simulink model "Candidacy_Exam_RR"  (R2023a)
settings: Solver=VariableStepAuto  StartTime=0  StopTime=1000  FixedStep=0.01  RelTol=1e-3
model workspace (MAT data in the model file):
  finalint = 0
  firstWarning = 1
  originalScenarioChecksum = '114339432DE22364D47BB28FC96DC10C'
undefined symbols (not defined in the file): Acceleration, ActorID, AngularVelocity, curvature, DefaultGear, Defined, DEND_B, DEND_S, DEND_T, direction, DiscIntNeverNeededParam, driving, Ego, EgoRefPose, gradbp, L, Lane, LF, LR, m, matlabshared, MAX_BRAKE, MAX_STEER, MAX_TORQUE, maxNumActors, MCAR, MIN_BRAKE, MIN_STEER, MIN_TORQUE, n, NUMD_B, NUMD_S, NUMD_T, Pitch, Pose, Position, psi_o, R, Roll, RRdamp, SceneInfo, session, sigbuilder_block, STEER_RATIO, stopSign_ID, Tdead, thetaRefs, TL_ID, TrackWidth, Ts, ts, User, Vdead, Velocity, WB, X_o, xRef2s, Y_o, Yaw, yRef2s
libraries: drivingscenarioandsensors x13, roadrunnerscenario x11, simulink x8, simulink_extras x5, drivingvehiclecontroller x2, trackingutilitieslib x2, robotalgslib x1, mpcadaslib x1, slpidlib x1, drivinglib x1, autolibshared x1, vehdynlibviscommon x1
(part 5 of 5)

== stateflow chart Candidacy_Exam_RR/Behavioural Planner/Chart ==
  settings: updateMethod=DISCRETE  sampleTime=Ts
  state Stationary
    en,du:
    VelCmd = 0;
    CurrentVelCmd = VelCmd;
    Navi = 0;
    Trans = 0;
    StopSim = 0;
    Tgap = 1;
    HoldBrake = 1;
    Braking = 0;
  state Navigation
    state RailCrossing [commented out]
      state Stop [commented out]
        en:
        VelCmd = 0;
        Braking = 1;
        CurrentVelCmd = VelCmd;
      state Approaching [commented out]
        en:
        Braking = 1;
        Tgap = 0;
        Trans = 0;
      state Transition [commented out]
        en:
        Tgap = 1;
        Trans = 1;
        Braking = 0;
        VelCmd = SceneSpeed;
        CurrentVelCmd = VelCmd;
      state ExitScene [commented out]
        en:
        ExitFlag = 1;
      (default) -> Navigation.RailCrossing.Approaching [commented out]
      Navigation.RailCrossing.Approaching -> Navigation.RailCrossing.Stop [commented out] : [D2S <= 6 && (RRCross == 1 || ObjectDist <= TransDist)]
      Navigation.RailCrossing.Transition -> Navigation.RailCrossing.Approaching [commented out] : [ObjectDist <= TransDist]
      Navigation.RailCrossing.Approaching -> Navigation.RailCrossing.Transition [commented out] : [RRCross == 0 && ObjectDist > TransDist && D2S <= 6]
      Navigation.RailCrossing.Stop -> Navigation.RailCrossing.Transition [commented out] : [RRCross == 0 && ObjectDist > TransDist]
      Navigation.RailCrossing.Approaching -> Navigation.RailCrossing.ExitScene [commented out] : [SceneID ~= 10]
      Navigation.RailCrossing.Transition -> Navigation.RailCrossing.ExitScene [commented out] : [SceneID == 0]
    state RoundAbout
      state Approaching
        en:
        Braking = 1;
        Trans = 0;
        Tgap = 0;
      state Stop
        en:
        VelCmd = 0;
        Braking = 1;
        CurrentVelCmd = VelCmd;
      state ExitScene
        en:
        ExitFlag = 1;
      state Transition
        en:
        Tgap = 1;
        Trans = 1;
        Braking = 0;
        VelCmd = SceneSpeed;
        CurrentVelCmd = VelCmd;
      (default) -> Navigation.RoundAbout.Approaching
      Navigation.RoundAbout.Approaching -> Navigation.RoundAbout.Stop [order 1] : [D2S <= 6]
      Navigation.RoundAbout.Stop -> Navigation.RoundAbout.Transition : [Clear2Go == 1]
      Navigation.RoundAbout.Approaching -> Navigation.RoundAbout.ExitScene [order 2] : [SceneID ~= 9]
      Navigation.RoundAbout.Transition -> Navigation.RoundAbout.ExitScene : [SceneID == 0]
    state DestCheck
      en,du:
      % dest reached?
      (default) -> (junction 47)
      (junction 47) -> (junction 48) [order 1] : [D2D < 2]
      (junction 47) -> (junction 49) [order 2] : {DestReached = 0;}
      (junction 48) -> (junction 50) : {DestReached = 1;}
      (junction 50) -> (junction 49) : {StopSim = 1;}
      (junction 49) -> (junction 51)
    state TrafficLight [commented out]
      note: Yellow light duration is 1s
      state Stop [commented out]
        en:
        Braking = 1;
        VelCmd = 0;
        CurrentVelCmd = VelCmd;
      state Approaching [commented out]
        en:
        Tgap = 0;
        Trans = 0;
        T2S = 0;
        %if TLstate(1,4) == 1
        Braking = 1;
        %else
        % ACC = 0;
        %end
      state DecisionOnYellow [commented out]
        en:
        T2S = D2S/EgoSpeed;
      state Transition [commented out]
        en:
        Trans = 1;
        Braking = 0;
        Tgap = 1;
        VelCmd = SceneSpeed;
        CurrentVelCmd = VelCmd;
      state ExitScene [commented out]
        en:
        ExitFlag = 1;
      DecisionOnYellow -> Navigation.TrafficLight.Approaching [commented out] : [T2S > 1.2]
      (default) -> Navigation.TrafficLight.Approaching [commented out]
      Navigation.TrafficLight.Approaching -> Navigation.TrafficLight.Stop [commented out] : [D2S <= 6]
      Navigation.TrafficLight.Stop -> Navigation.TrafficLight.Transition [commented out] : [TLstate(1,4) == 3 && ObjectDist > TransDist]
      Navigation.TrafficLight.Transition -> Navigation.TrafficLight.Approaching [commented out] : [TLstate(1,4) == 1  || ObjectDist < TransDist]
      Navigation.TrafficLight.Approaching -> Navigation.TrafficLight.Transition [commented out] : [TLstate(1,4) == 3 && ObjectDist > TransDist]
      Navigation.TrafficLight.Approaching -> Navigation.TrafficLight.ExitScene [commented out] : [SceneID ~= 8]
      Navigation.TrafficLight.Transition -> DecisionOnYellow [commented out] : [TLstate(1,4) == 2]
      DecisionOnYellow -> Navigation.TrafficLight.Transition [commented out] : [T2S <= 1.2]
      Navigation.TrafficLight.Transition -> Navigation.TrafficLight.ExitScene [commented out] : [SceneID == 0]
    state Drive
      en :
      HoldBrake = 0;
      VelCmd = RoadSpeed;
      CurrentVelCmd = VelCmd;
      ExitFlag = 0;
    state Go
      en:
      VelCmd = RoadSpeed;
      CurrentVelCmd = VelCmd;
      Trans = 0;
      ExitFlag = 0;
      Braking = 0;
      HoldBrake = 1;
    state StopSign
      state StoptSign4way
        state CheckInt
          du:
          % stopped?
          % ss priority?
        state CheckSS
          % stopped?
          % ss priority?
        state Transition
          en:
          % stay here while trans?!
          % while ~crossedLimitLine of TargetLane
          Trans = 1;
          Braking = 0;
          Tgap = 1;
          VelCmd = SceneSpeed;
          CurrentVelCmd = VelCmd;
        state ExitScene
          en:
          ExitFlag = 1;
        (default) -> Navigation.StopSign.StoptSign4way.CheckSS
        Navigation.StopSign.StoptSign4way.CheckSS -> Navigation.StopSign.StoptSign4way.CheckInt : [EgoSpeed < VelStop]
        Navigation.StopSign.StoptSign4way.CheckInt -> Navigation.StopSign.StoptSign4way.Transition : [egoSSPriority == 1 && Clear2Go == 1]
        Navigation.StopSign.StoptSign4way.Transition -> Navigation.StopSign.StoptSign4way.ExitScene : [SceneID == 0 && after(2,sec)]
      state SStype
        state Approaching
          en:
          %VelCmd = ApproachingSpeed;
          Braking = 1;
          Trans = 0;
          Tgap = 0;
        state Stop
          en:
          VelCmd = 0;
          Braking = 1;
          CurrentVelCmd = VelCmd;
        Navigation.StopSign.SStype.Stop -> 410 [order 1] : [numSS == 4]
        (default) -> Navigation.StopSign.SStype.Approaching
        Navigation.StopSign.SStype.Approaching -> Navigation.StopSign.SStype.Stop : [D2S <= 15]
        Navigation.StopSign.SStype.Stop -> 414 [order 2] : [numSS == 2]
      state StopSign2way
        state CheckInt
          en:
          VelCmd = 0;
          HoldBrake = 1;
          CurrentVelCmd = VelCmd;
        state CheckSS
          % stopped?
          % ss priority?
        state Transition1
          en:
          % stay here while trans?!
          % while ~crossedLimitLine of TargetLane
          Trans = 1;
          Braking = 0;
          HoldBrake = 0;
          Tgap = 1;
          VelCmd = SceneSpeed;
          CurrentVelCmd = VelCmd;
        state ExitScene1
          en:
          ExitFlag = 1;
        (default) -> Navigation.StopSign.StopSign2way.CheckSS
        Navigation.StopSign.StopSign2way.CheckSS -> Navigation.StopSign.StopSign2way.CheckInt : [EgoSpeed < VelStop]
        Navigation.StopSign.StopSign2way.CheckInt -> Transition1 : [egoSSPriority == 1 && ToAClearance == 1]
        Transition1 -> Navigation.StopSign.StopSign2way.CheckInt [order 2] : [ToAClearance == 0]
        Transition1 -> ExitScene1 [order 1] : [SceneID == 0 && after(1,sec) && egoExit == 1]
      (default) -> SStype
      416 -> StoptSign4way
      411 -> StopSign2way
    Go -> RailCrossing [commented out] : [SceneID == 10]
    Drive -> RailCrossing [commented out] : [SceneID == 10]
    RailCrossing -> Go [commented out] : [ExitFlag == 1]
    Go -> RoundAbout [order 2] : [SceneID == 9]
    Drive -> RoundAbout [order 1] : [SceneID == 9]
    RoundAbout -> Go : [ExitFlag == 1]
    (default) -> DestCheck
    Drive -> TrafficLight [commented out] : [SceneID == 8]
    DestCheck -> Drive : [DestReached == 0]
    Go -> TrafficLight [commented out] : [SceneID == 8]
    Drive -> DestCheck [order 3] : [D2D < 2]
    TrafficLight -> Go [commented out] : [ExitFlag == 1]
    Drive -> StopSign [order 2] : [SceneID == 7]
    StopSign -> Go : [ExitFlag == 1]
    Go -> DestCheck [order 1] : [SceneID == 0]
    Go -> StopSign [order 3] : [SceneID == 7]
  (default) -> Stationary
  Stationary -> Navigation : [Navigate == 1]
  Navigation -> Stationary : [Navigate == 0 || DestReached == 1]
  data: TLstate input; numSS input; egoExit input; ToAClearance input; TransDist input; ApproachingSpeed input; EgoSpeed input; ObjectDist input; SceneSpeed input; SDist input; RRCross input; D2S input; DestReached local; Navigate input; ExitFlag local; D2D input; Clear2Go input; RoadSpeed input; CurrentVelCmd local; Navi local; VelCmd output; HoldBrake output; SceneID input; Tgap output; Trans output; StopSim output; Braking output; T2S local; VelStop input; egoSSPriority input

== matlab function Candidacy_Exam_RR/Behavioural Planner/MATLAB Function ==
  data: u input; y output
function y = fcn(u)

y = u;

== matlab function Candidacy_Exam_RR/Subsystem/Function-Call Subsystem/MATLAB Function1 ==
  data: EgoPosition input; MIOPos input; curvature input; MIOVel input; V_i input; xd output; yd output; laneL input; laneR input; V_desired input; LCinProgress output
function [xd,yd,LCinProgress] = traj(EgoPosition,MIOPos,curvature,MIOVel, V_i, laneL, laneR, V_desired)
Vx_i =0;Vx_f=0;Vy_i=0;Vy_f=0;Ax_i=0;Ax_f=0;Ay_i=0;Ay_f=0;T_i=0;T_f=0;V_f=0;A_f=0;x_set=0;y_set=0;theta4=0;

P = zeros(6,6);
% xq = zeros(1,size(RefPath,1)); yq = zeros(1,size(RefPath,2));
EgoPosition(1,2)=-EgoPosition(1,2);
x_init= EgoPosition(1,1)+2; y_init = EgoPosition(1,2)-2;
% xq = RefPath(:,1)'; 
% yq = RefPath(:,2)';
num_foc_t = 98;
V_max= V_desired; ad_n=0; vd_n=MIOVel; wd_n=vd_n*curvature;
lane_width = 3.6 * (laneL-laneR); % +1 if left of current lane and -1 if right of current lane(rahul flipped)
xd = zeros(num_foc_t+1,1); 
yd = zeros(num_foc_t+1,1);
xf =0; 
yf = 0;

    %xf = [EgoPosition(1,1)+ MIOPos(1) ]; yf = [ EgoPosition(1,2)+ MIOPos(2) + lane_width];  
    xf = [EgoPosition(1,1)+ 20 ]; yf = [EgoPosition(1,2)+ lane_width]; % 80
    V_f = V_max;
    W_f = V_f*curvature;
    A_f = 0;

    %dist2crash = sqrt((x_init-MIOPos(1))^2+(y_init-MIOPos(2))^2);
    %dist2crash = 40;
    %T_f = abs(dist2crash/(MIOVel-V_i));
    T_f = 3;
    P = [1, T_i, T_i^2, T_i^3, T_i^4, T_i^5;
         0, 1, 2*T_i, 3*T_i^2, 4*T_i^3, 5*T_i^4;
         0, 0, 2, 6*T_i, 12*T_i^2, 20*T_i^3;
         1, T_f, T_f^2, T_f^3, T_f^4, T_f^5;
         0, 1, 2*T_f, 3*T_f^2, 4*T_f^3, 5*T_f^4;
         0, 0, 2, 6*T_f, 12*T_f^2, 20*T_f^3];

%     mtang4 = (yq(1,index+2)-yq(1,index+1))/(xq(1,index+2)-xq(1,index+1));

    Vx_i = vd_n*cos(theta4); 
    Vy_i = vd_n*sin(theta4); 
    Ax_i = ad_n*cos(theta4)-vd_n*sin(theta4)*wd_n; 
    Ay_i = ad_n*sin(theta4)+vd_n*cos(theta4)*wd_n;

%     if(xq(index+2)-xq(index+1)<0)
%         theta_4 = pi + atan(mtang4);
%     else
%         theta_4 = atan(mtang4);
%     end

    theta_4 =0;
    Vx_f = V_f*cos(theta_4); % curvature angle
    Vy_f = V_f*sin(theta_4);
    Ax_f = A_f*cos(theta_4)-V_f*sin(theta_4)*W_f;
    Ay_f = A_f*sin(theta_4)+V_f*cos(theta_4)*W_f;

    g1 = [x_init; Vx_i; Ax_i; xf; Vx_f; Ax_f];
    g2 = [y_init; Vy_i; Ay_i; yf; Vy_f; Ay_f];

    a_coeff = P\g1;
    b_coeff = P\g2;
    
    td = T_i;
    scatter(x_init,y_init,'go')
    hold on; 
    scatter(xf,yf,'ro')
    hold on;
    
    for f = 1:(num_foc_t+1)
        xd(f,1) = [1,td,td^2,td^3,td^4,td^5]*a_coeff 
        yd(f,1) = [1,td,td^2,td^3,td^4,td^5]*b_coeff
        td = td + (T_f - T_i)/num_foc_t;
        scatter(xd(f,1),yd(f,1),'y.');
    end

LCinProgress = 1;

% hold on;
end

== matlab function Candidacy_Exam_RR/Behavioural Planner/StopSignPriority ==
  settings: updateMethod=DISCRETE
  data: ToAClearance output; SDist input; D2S input; ObjTracks input; egoSSPriority output; SceneTracks input; egoPose input; egoSpeed input; numSS output; VelStop input; WB input; d output; flag input; flag output; midpoint input; midpoint output; egoExit output; egoEnter input; egoEnter output
function [ToAClearance, egoSSPriority, numSS, d, flag, midpoint, egoExit, egoEnter]  = StopSignPriority(SDist, D2S, ObjTracks, SceneTracks, egoPose, egoSpeed, VelStop, WB, flag, midpoint, egoEnter)
% calculate covariance matrix outside, input to this block is modified with final, unique detections

egoPose(2) = -egoPose(2);
egoPose(3) = -egoPose(3);
persistent SSPriority C1x C2y C3x C4y
% find stop signs + one of 2way or 4way or T-junction

% find number of signs (until we reach 0 valued columns)
numSS = 0;
for j = 1:length(SceneTracks(1,:))
    if any(SceneTracks(:,j))
        numSS = numSS + 1;
    end
end

% find number of cars
numCars = 0;
for j = 1:length(ObjTracks(1,:))
    if any(ObjTracks(:,j))
        numCars = numCars + 1;
    end
end


egoSSPriority = 1;
ToAClearance = 1;
% tempPriority = zeros(numCars+1,1);
d = zeros(10, 5); % distance, velocity, time, location (wrt ego), exit (leaving ints)
Objang = zeros(10, 1);
% priorityTable = zeros(numCars+1, 5);
egoExitang = egoPose(3) - atan2d(midpoint(2)-egoPose(2),midpoint(1)-egoPose(1)); % 0 deg = straight , + = right
egoExitdist = sqrt((midpoint(2)-egoPose(2))^2+(midpoint(1)-egoPose(1))^2);

if abs(egoExitang) >= 135 && egoExitdist >= 1 && egoEnter == 1
    d(1,5) = 1; % left the ints
    egoEnter = 0;
    flag = 0;
elseif abs(egoExitang) >= 135 && egoExitdist <= 10
    d(1,5) = 1;
end
egoExit = d(1,5);


if D2S <= SDist || egoEnter == 1

    % [~, index] = min(abs(SceneTracks(1,:)'));
    if numSS > 0

        Vmd = [-egoSpeed*sind(egoPose(3)), egoSpeed*cosd(egoPose(3))];
        rot = [cosd(egoPose(3)) -sind(egoPose(3)); sind(egoPose(3)) cosd(egoPose(3))];

        % intersection region
        if flag == 0
            C1x = min(SceneTracks(1, 1:numSS)) - (WB + 3);
            C2y = min(SceneTracks(3, 1:numSS)) - (WB + 3);
            C3x = max(SceneTracks(1, 1:numSS)) + (WB + 3);
            C4y = max(SceneTracks(3, 1:numSS)) + (WB + 3);
            C1 = rot*[C1x; C2y] + egoPose(1:2)';
            C2 = rot*[C3x; C4y] + egoPose(1:2)';
            midpoint = (C1+C2)./2;
            % midpoint = [2*egoPose(1)-C4y-C2y; 2*egoPose(2)+C1x+C3x]./2;
        %   scatter(-SceneTracks(3,:)+egoPose(1),SceneTracks(1,:)+egoPose(2),'blue','filled')   
            scatter(midpoint(1), midpoint(2), 'blue', 'filled')
            rectangle('Position',[egoPose(1)-C4y egoPose(2)+C1x abs(C4y-C2y) abs(C3x-C1x)])
            flag = C1x;
        end

       
        midpoint_ego = rot'*(midpoint - egoPose(1:2)');
        % loop through num of cars (j)
    
        d(1,1) = sqrt((midpoint(1) - egoPose(1))^2 + (midpoint(2) - egoPose(2))^2);
        d(1,2) = egoSpeed;
        d(1,3) = d(1,1)/d(1,2);     %add ego TOA
        d(1,4) = 4; % 4 is the location of the ego vehicle itself
        
        if d(1,1) <= 3
            ToAThreshold = 1;
        else
            ToAThreshold = 3;
        end

        if d(1,1) <= flag
            egoEnter = 1;
        end

    
        % loop through signs (vectorized)
        % if smallest dist 
        % d(:,3) -> TOA = v/dist
    
        if numCars > 0
            for k = 1:numCars
                d(k+1,1) = sqrt((midpoint_ego(2)-ObjTracks(3,k))^2+(midpoint_ego(1)-ObjTracks(1,k))^2); %sqrt((midpoint(1) - (-ObjTracks(3,k)+egoPose(1)))^2 + (midpoint(2) - (ObjTracks(1,k)+egoPose(2)))^2); 
                d(k+1,2) = sqrt((Vmd(1) - ObjTracks(2,k))^2 + (Vmd(2) - ObjTracks(4,k))^2);
                d(k+1,3) = d(k+1,1)/d(k+1,2); % TOA of other cars
                Objang(k) = atan2d(ObjTracks(1,k), -ObjTracks(3,k));
                                
                % Identify cars location (direction) wrt ego
                if Objang(k) <= 60
                    d(k+1,4) = 1; % 1 = E, 2 = N, 3 = W
                elseif Objang(k) > 60  && Objang(k) < 120
                    d(k+1,4) = 2; % 1 = E, 2 = N, 3 = W
                elseif Objang(k) >= 120
                    d(k+1,4) = 3; % 1 = E, 2 = N, 3 = W
                end

                % Identifying leaving cars
                
                ActorHeading = atan2d(ObjTracks(2,k) - Vmd(1), -ObjTracks(4,k) - Vmd(2));
                actorExitang = ActorHeading - atan2d(midpoint_ego(1)-ObjTracks(1,k),midpoint_ego(2)+ObjTracks(3,k)); % 0 deg = straight , + = right
                %actorExitdist = sqrt((midpoint_ego(2)-ObjTracks(3,k))^2+(midpoint_ego(1)-ObjTracks(1,k))^2);
                

                if abs(actorExitang) >= 135 && d(k+1,1) >= 10 
                    d(k+1,5) = 1; % left the ints
                else
                    d(k+1,5) = 0; % did not leave
                end

    
            end
    
            if numSS == 4 
                % Assign priorities based on rank TOA #1, before vehicle stops
                % d1 = d(d(:,1)~=0,:);
                [car, SSPriority] = sort(d(d(:,1)~=0 & d(:,5)==0));
                % priorityTable(:, 1:2) = [car, priority];
        
                tempPriority = find(SSPriority == 1); % ego SS priority
                % for idx = 1:nn(vv<vv(find(nn==1)))
                % 
                % end
        
                egoSSPriority = tempPriority(1);
    
            elseif numSS == 2
                [car, SSPriority] = sort(d((d(:,4)==2 | d(:,4)==4) & d(:,5)==0));
                tempPriority = find(SSPriority == 1); % ego SS priority
                egoSSPriority = tempPriority(1);
                ToAClearance = double(all(d(d(:,1)~=0 & d(:,5)==0 & d(:,4)~=4,3) > ToAThreshold));

            elseif numSS == 1
                [car, SSPriority] = sort(d((d(:,4)==2 | d(:,4)==4) & d(:,5)==0));
                tempPriority = find(SSPriority == 1); % ego SS priority
                egoSSPriority = tempPriority(1);
                ToAClearance = double(all(d(d(:,1)~=0 & d(:,5)==0 & d(:,4)~=4,3) > ToAThreshold));

            end
    
        end
    end
    
    
    
    
    % if egoSpeed <= VelStop
    %     if SSPriority ~= 1
    %         % for all vehicles with higher priority
    %         % provide indicator signals to identify conflicts
    %         % check indicator signs/conflicts and update priority based on that
    %         % code to define leavingScene for other vehicles:
    %         % update priority table
    % 
    %     end
    % end
    
    
    
    

% elseif egoExit == 0
    

end

== matlab function Candidacy_Exam_RR/Behavioural Planner/MATLAB Function1 ==
  data: EgoLength input; TransDist output; IntDist input
function TransDist = IntersectionClearanceDist(EgoLength,IntDist)

TransDist = IntDist + EgoLength;

== matlab function Candidacy_Exam_RR/Subsystem/Turns LC in prog off ==
  data: u input; y output
function y = fcn(u)

persistent counter;
persistent input_high;

if isempty(counter)
    counter = 0;
end

if isempty(input_high)
    input_high = false;
end

if u ~= 0
    input_high = true;
end

if input_high && counter < 100
    y = u;
    counter = counter + 1;
else
    y = 0;
end

== matlab function Candidacy_Exam_RR/Controllers/Longitudinal Controllers/Subsystem/Distance to Traffic Sign ==
  data: currentDistanceTravelled input; relativeDistanceToScene output; signLatPose input; signLongPose input; ego_vel input; cumulativeDistance input; CurrentPose input; RefXY input; sceneDistance output; sceneDistance input; signPose output
function [relativeDistanceToScene, sceneDistance,signPose] = fcn(currentDistanceTravelled, signLatPose, signLongPose, ego_vel, cumulativeDistance, CurrentPose, RefXY, sceneDistance)

signPose=[40 40];
if signLongPose ~= 0
    % X front side of car, Y right side of car

    thetaSS = atan2d(signLongPose, signLatPose);

    
    beta = thetaSS+CurrentPose(3) - 90;
    alphaVector = norm([signLongPose, signLatPose]);
    xSS = alphaVector*cosd(beta);
    ySS = alphaVector*sind(beta);
    signPose = [xSS + CurrentPose(1), ySS + CurrentPose(2)];
    % signPose = [xSS - CurrentPose(2), ySS + CurrentPose(1)]; % y is x , x is -y

    
    %%%
    % signPose = [RefXY(end,1) RefXY(end,2)];

    distance = zeros(length(RefXY),1);
    for j = 1:length(RefXY)
        distance(j) = norm(signPose(1:2) - RefXY(j,1:2));
    end
    
    [~, ind] = mink(distance,2);
    
    if ind(1) > ind(2)
        ind = [ind(2); ind(1)];
    end

    signPoseOnPath = [0 0];
    m = 0; mm = 0; b = 0; bb = 0;
    m = (RefXY(ind(1),2) - RefXY(ind(2),2))/(RefXY(ind(1),1) - RefXY(ind(2),1));
    if m == 1e6
        signPoseOnPath = [RefXY(ind(1),1) signPose(2)];
    elseif m == 1e-6
        signPoseOnPath = [signPose(1) RefXY(ind(1),2)];
    else
        b = RefXY(ind(1),2) - m*RefXY(ind(1),1);
        mm = -1/m;
        bb = signPose(2) - mm*signPose(1);
        signPoseOnPath(1:2) = [(b-bb)/(mm-m) m*((b-bb)/(mm-m))+b];     
    end


    sceneDistance = cumulativeDistance(ind(1)) + norm(RefXY(ind(1),1:2) - signPoseOnPath(1:2)); % Distance to scene/sign, local origin
    relativeDistanceToScene = sceneDistance - currentDistanceTravelled - (2.6850 + 1); % Longitudinal Distance from Ego Vehicle to Scene
    %%%
else

    relativeDistanceToScene = sceneDistance - currentDistanceTravelled - (2.6850 + 1);
end

end

== matlab function Candidacy_Exam_RR/Controllers/Longitudinal Controllers/MATLAB Function ==
  data: x output; u input; y output
function [x, y] = fcn(u)
y = 0; x = 0;
y = u(1,1);
x = u(3,1);

== matlab function Candidacy_Exam_RR/Environment & Data/Roadrunner Port/ENU to NWD/2D RefWaypoints ==
  data: u input; y output; initialYaw output
function [y, initialYaw] = fcn(u)

y = u(:,1:2);
initialYaw = atan2(u(2,2) - u(1,2),u(2,1) - u(1,1));
end

== matlab function Candidacy_Exam_RR/Environment & Data/Roadrunner Port/ENU to NWD/MATLAB Function ==
  data: traj input; destination_traj output; last_idx output; Initial_traj output
function [destination_traj,last_idx,Initial_traj] = DestinationPoint(traj)

last_idx = 1;

for i=1:length(traj)
    if norm(traj(i,1:2)) == 0
        last_idx = i-1;
        break
    end
end

destination_traj = traj(last_idx,1:2);
Initial_traj = traj(1,1:2);

end

== matlab function Candidacy_Exam_RR/Subsystem/PathPlanner/MATLAB Function3 ==
  settings: updateMethod=DISCRETE
  data: out output; check output; Xref input; Yref input; xd input; yd input; LC input; current_pos input; d2f input; dcheck output
function [out,check,dcheck]  = PathPlanning(Xref, Yref, xd, yd, LC, current_pos, d2f)

persistent output_matrix
persistent lc_triggered

if isempty(lc_triggered)
lc_triggered = false;
end

%lc_triggered=0;
%if isempty(hold_output)
  %  hold_output = false;
%end


if isempty(output_matrix)
    output_matrix = [Xref(:), Yref(:)];
    out = [Xref(:), Yref(:)];
else
    out = output_matrix;
end

if LC && ~isempty(xd) && ~isempty(yd)
    output_matrix = [xd(:), yd(:)];
    lc_triggered=true;
       
end

check=lc_triggered;
dcheck=output_matrix;
%out=output_matrix;

if lc_triggered && d2f < 5 %&& ~isempty(output_matrix) %&& ~hold_output
    %Yout = Yref(:);
    if current_pos > 0
        Xout = Xref(:);
        Yout = Yref + 3.6;
    else
        Xout = Xref(:);
        Yout = Yref;
    end
    output_matrix = [Xout, Yout];
    out=output_matrix;
    lc_triggered=false;
    %hold_output = true;
end

out=output_matrix;




%if ~LC && ~isempty(output_matrix) && lc_triggered
    %hold_output = false;
    %lc_triggered=false;
%end

end

== stateflow chart Candidacy_Exam_RR/Behavioural Planner/Routing ==
  state InitialRoute
    en:
    NewRoute = 0;
  state Rerouting
    en:
    NewRoute = 1;
  (default) -> InitialRoute
  InitialRoute -> Rerouting : [ReRoute == 1]
  Rerouting -> InitialRoute : [ReRoute == 0]
  data: ReRoute input; NewRoute output

== matlab function Candidacy_Exam_RR/Environment & Data/Roadrunner Port/ENU to NWD/MATLAB Function1 ==
  data: traj input; trajectory_way output
function trajectory_way = fcn(traj)

last_idx = 1;

for i=1:length(traj)
    if norm(traj(i,1:2)) == 0
        last_idx = i-1;
        break
    end
end

trajectory_way = zeros(150,2);

for j = 1:last_idx
    trajectory_way(j,:) = traj(j,1:2);
end


for k = (last_idx+1):100
    trajectory_way(k,:) = trajectory_way(last_idx,:);
end

== matlab function Candidacy_Exam_RR/Environment & Data/Roadrunner Port/ENU to NWD/MATLAB Function2 ==
  data: u input; y output; y1 output
function [y,y1] = fcn(u)

y = u(:,1);
y1=u(:,2);

== matlab function Candidacy_Exam_RR/Environment & Data/Roadrunner Port/Initial State/Initialize State/Calculate Initial States/Calculate Initial States ==
  data: egoRuntime input; egoInitialState output Bus: BusVehicleInfo
function egoInitialState = getInitialState(egoRuntime)
%getInitialState calculates initial conditions of the vehicle

% Calculate velocity
velocity = norm(egoRuntime.ActorRuntime.Velocity,2);
% Get Transformation matrix
transformationMatrix = egoRuntime.ActorRuntime.Pose;
% Get pose information
x = transformationMatrix(1,4);
y = transformationMatrix(2,4);
yaw = atan2d(-transformationMatrix(1,2), ...
            transformationMatrix(1,1));
% Pack the initial states
egoInitialState = struct('CurrPose', [y, -x, yaw], ...
    'CurrVelocity', velocity, ...
    'CurrYawRate', 0, ...
    'CurrSteer',0, ...
    'Direction',1);

== matlab function Candidacy_Exam_RR/Environment & Data/Sensors & Perception/Tracking1/MATLAB Function ==
  data: u input; y output; y1 output
function [y,y1] = fcn(u)
TracksNum = u.NumTracks;
y = zeros(20,1);
for k = 1:TracksNum
    y(k) = u.Tracks(k).ObjectAttributes.TargetIndex;
end
y1 = u.Tracks(1).ObjectAttributes.TargetIndex;

== matlab function Candidacy_Exam_RR/Environment & Data/Roadrunner Port/MATLAB Function ==
  data: ActorsIn input; EgoVeh input; EgoRefActors output Bus: BusWorldToVehicleActors
function EgoRefActors  = GlobaltoEgoRefConv(ActorsIn,EgoVeh)
%ActorsOut = Simulink.Bus;
ActorsOut = ActorsIn;
numActors = length(ActorsIn.Actors);
for k = 1:numActors
    actorOut = driving.scenario.targetsToEgo(ActorsIn.Actors(k),EgoVeh);
    ActorsOut.Actors(k).ActorID             = actorOut.ActorID;
    ActorsOut.Actors(k).Position            = actorOut.Position;
    ActorsOut.Actors(k).Velocity            = actorOut.Velocity;
    ActorsOut.Actors(k).Roll                = actorOut.Roll;
    ActorsOut.Actors(k).Pitch               = actorOut.Pitch;
    ActorsOut.Actors(k).Yaw                 = actorOut.Yaw;
    ActorsOut.Actors(k).AngularVelocity    = actorOut.AngularVelocity;
end
EgoRefActors = ActorsOut;
end
